simulink model "TestCinematicaz_Primera_Parte"  (R2023b)
settings: Solver=FixedStepDiscrete  StartTime=0.0  StopTime=10  FixedStep=0.01  RelTol=1e-3  EnableMultiTasking=on
model workspace (MAT data in the model file):
  d = 0.195
settings Model: ExtModeTrigDuration=2  Creator=marqu  LastModifiedBy=marqu
settings OptimizationCC: EnhancedBackFolding=on  PassReuseOutputArgsAs=Individual arguments  ZeroExternalMemoryAtStartup=off  ZeroInternalMemoryAtStartup=off  MaxStackSize=64  OptimizeBlockOrder=speed  DifferentSizesBufferReuse=on  EfficientTunableParamExpr=on
settings DebuggingCC: ParameterTunabilityLossMsg=error
settings HardwareCC: ProdBitPerInt=16  ProdBitPerPointer=16  ProdBitPerSizeT=16  ProdBitPerPtrDiffT=16  ProdLargestAtomicFloat=None  ProdWordSize=8  ProdHWDeviceType=Atmel->AVR
settings SFSimCC: MATLABDynamicMemAlloc=off
settings RTWCC: Description=Embedded Coder  SystemTargetFile=ert.tlc  HardwareBoard=Arduino Mega 2560  TemplateMakefile=ert_default_tmf  Toolchain=Arduino AVR  BuildConfiguration=Faster Runs
settings CodeAppCC: ForceParamTrailComments=on  IgnoreCustomStorageClasses=off  OperatorAnnotations=on  SimulinkDataObjDesc=on  SFDataObjDesc=on  InsertBlockDesc=on
settings ERTTargetCC: SupportContinuousTime=on  SupportVariableSizeSignals=on  ExtModeTransport=3  ExtModeStaticAlloc=on  ExtModeAutomaticAllocSize=off  ExtModeStaticAllocSize=2048  ExtModeMexFile=ext_xcp  ExtModeIntrfLevel=Level2 - Open

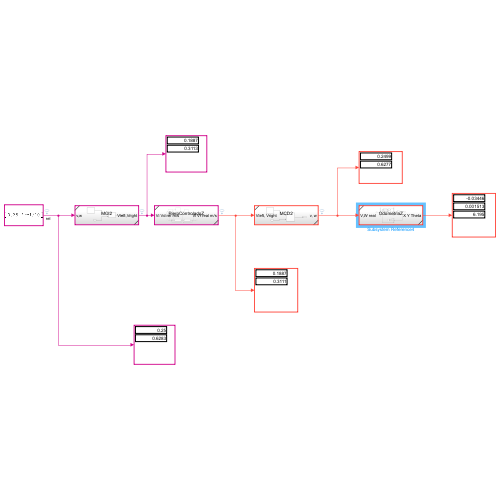
[thumbnail: Simulink's stored preview of the top-level diagram]
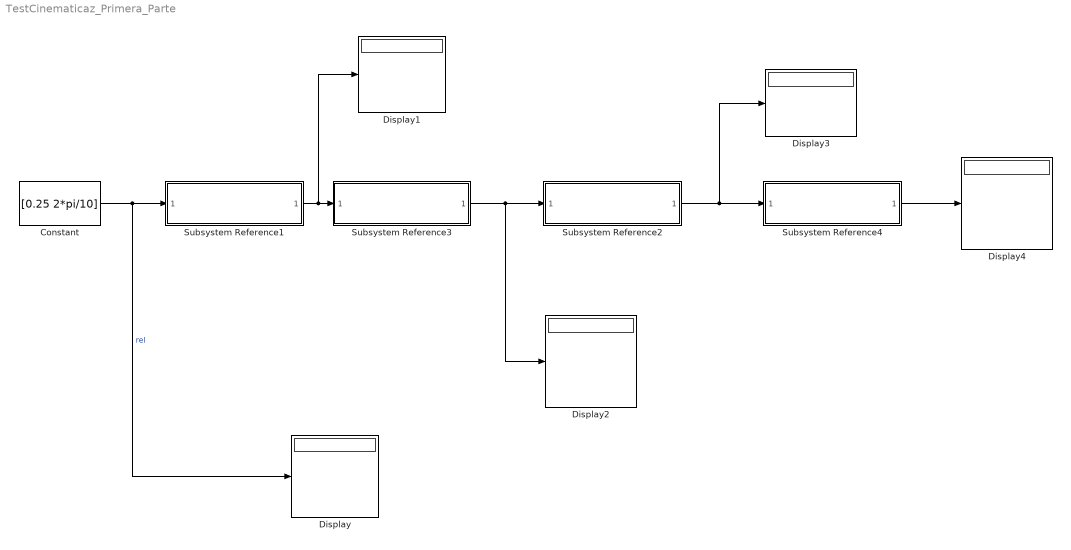
== system TestCinematicaz_Primera_Parte ==
  Constant : Constant  Value=[0.25 2*pi/10]  VectorParams1D=off
  Display{,1..4} (5 alike) : Display
  Subsystem Reference1 : Subsystem  ReferencedSubsystem=MCI2
  Subsystem Reference2 : Subsystem  ReferencedSubsystem=MCD2
  Subsystem Reference3 : Subsystem  ReferencedSubsystem=PieroControladoZ
  Subsystem Reference4 : Subsystem  ReferencedSubsystem=OdometriaZ
  wires:
  Subsystem Reference1/1 -> Display1/1, Subsystem Reference3/1
  Subsystem Reference2/1 -> Display3/1, Subsystem Reference4/1
  Subsystem Reference3/1 -> Display2/1, Subsystem Reference2/1
  Constant/1 -> Display/1, Subsystem Reference1/1  "rel"
  Subsystem Reference4/1 -> Display4/1
